simulink model "BikeRLAgent"  (R2023b)
settings: Solver=VariableStepAuto  StartTime=0.0  StopTime=inf  RelTol=1e-3
values from neighbouring files (symbols this model uses):
  angleFF = (lambda)    [config.m]
  angleRF = angleRF * (180/pi)    [config.m]
  b_contact_RW = 2e3    (= 2000)    [config.m]
  C_F_alpha = 1e3    (= 1000)    [config.m]
  C_F_kappa = 1e3    (= 1000)    [config.m]
  CM_phi = 0.3    [config.m]
  Dtheta0 = v0 / radiusRW    (= 0)    [config.m]
  Dtheta0_FW = v0 / radiusFW    (= 0)    [config.m]
  epsilon = 1e-2    (= 0.01)    [config.m]
  g = 9.81    [config.m]
  isoCameraAimX = (1/2)*w + 0.75    (= 1.267)    [config.m]
  isoCameraX = -2    [config.m]
  isoCameraY = -1.0    (= -1)    [config.m]
  isoCameraZ = -2*w    (= -2.068)    [config.m]
  k_contact_FW = 1e5    (= 100000)    [config.m]
  k_contact_RW = 1e5    (= 100000)    [config.m]
  lengthFF = frontHinge / (sind(lambda))    [config.m]
  lengthRF = sqrt((w-frontHinge)^2 + adj^2)    [config.m]
  lengthRW = 0.03    [config.m]
  massRW = 2    [config.m]
  max_cte = 7    [config.m]
  max_lean = 60    [config.m]
  max_positive_vel_error = 3    [config.m]
  max_rw_t = 20.0    (= 20)    [config.m]
  max_steer_t = 2.0    (= 2)    [config.m]
  max_steering = 70    [config.m]
  mB = 15    [config.m]
  mH = 5    [config.m]
  radiusFW = 0.325    [config.m]
  radiusRW = 0.32    [config.m]
  ref_v = ref_v_lims(1) + (ref_v_lims(2) - ref_v_lims(1))*rand(1,1)    [ResetFcn.m]
  sigma = 0.12    [config.m]
  topViewX = -4.5*w    (= -4.653)    [config.m]
  topViewY = 0*w    (= 0)    [config.m]
  topViewZ = 1*w    (= 1.034)    [config.m]
  xPla = 3e3    (= 3000)    [config.m]
  yPla = 3e3    (= 3000)    [config.m]
  zPla = 0.01    [config.m]
undefined symbols (not defined in the file or in its folder): Cylinder, Parts_Lib, ref_theta, ref_x, ref_y, X, Y, Z
libraries: sm_lib x78, nesl_utility x32, vrlib x14, simulink x6, rllib x1
(part 1 of 4)
Description:
  | Bicycle Simator was developed as a requirement for my Thesis, supervised by Alen Turnwald (MSc) at the Institute of Control Systems, TU Kaiserslautern.
  | 
  | More details on the theory can be found for the tire models at:
  | 
  | [1] De Vries , E J H. ; Den Brok , J F A.: Assessing slip of a rolling disc and the implementation of a tyre model in the benchmark bicycle. (2010), S. 20–22
  | 
  | [2] denBrok , J.F.A: A SimMechnaics Motorcycle Tyre Model for Real Time Purposes , TU Delft, Diplomarbeit
  | 
  | [3] Pacejka , H.B.: Tyre and Vehicle Dynamics.
  | 
  | [4] Maurice , J.P ; Pacejka , H.B: Relaxation length behavior of tyres. In: Vehicle System Dynamics Supplement S1 (1997), Nr. 27, S. 339–342. http://dx.doi.org/10.1080/00423119708969668. – DOI10.1080/00423119708969668
  | 
  | The bicycle modes are simulated according to:
  | 
  | [1] Meijaard , J.P. ; Papadopoulos , Jim M. ; Ruina , Andy ; Schwab , A.L.: Linearized dynamics equations for the balance and steer of a bicycle: a benchmark and review. In:
  | Proceedings of the Royal Society A: Mathematical, Physical and Engineering Sciences (2007). http://dx.doi.org/10.1098/rspa.2007.1857 . – DOI
  | 10.1098/rspa.2007.1857. – ISBN 1364–5021
  | 
  | For any suggestions or questions on the simulator, please contact me at : rzwn.hmd@gmail.com
  | 
  | For more info on the project at TU Kaiserslautern, please contact Alen through the website https://www.eit.uni-kl.de/liu/
settings Model: Creator=Rizwan Ahmed  LastModifiedBy=Asus
settings SolverCC: AlgebraicLoopSolver=TrustRegion
settings DebuggingCC: UnconnectedInputMsg=warning  UnconnectedOutputMsg=warning  UnconnectedLineMsg=warning  ArithmeticOperatorsInVariantConditions=warning
settings ModelReferenceCC: EnableRefExpFcnMdlSchedulingChecks=on
settings SFSimCC: SimUseLocalCustomCode=off  CustomCodeUndefinedFunction=UseInterfaceOnly
settings RTWCC: RTWUseLocalCustomCode=off
settings SimscapeCC: SimscapeLogType=all
settings ExplorerConfigSet: SimMechanicsOpenEditorOnUpdate=off  InternalSimMechanicsExplorerSettings="<ExplorerConfiguration><canonicalview>default</canonicalview><AnimationSetting><BasePlaybackSpeed>1.0</BasePlaybackSpeed><PlaybackSpeedFactor>1.0</PlaybackSpeedFactor></AnimationSetting><TilePanel><TileInfo><Tiles Columns=\"2\" Count=\"2\" Rows=\"1\"><Column Weight=\"0.492\"/><Column Weight=\"0.508\"/><Row Weight=\"1\"/><Tile Height=\"1\" Width=\"1\" X=\"0\" Y=\"0\"/><Tile Height=\"1\" Width=\"1\" X=\"1\" Y=\"0\"/></Tiles></TileInfo><SceneInfo><SceneViewer><BGColor><R>0.60000002384185791</R><G>0.60000002384185791</G><B>0.60000002384185791</B></BGColor><Camera><DoPerspective>on</DoPerspective><Position><X>40.0793484798167796</X><Y>-430.838153346124784</Y><Z>1.66080398163320275</Z></Position><Center><X>36.3390777502768501</X><Y>-431.839381200916819</Y><Z>0.597722304368772495</Z></Center><Up><X>0</X><Y>0</Y><Z>1</Z></Up><ViewLimDist>1</ViewLimDist><YLim>0.466307658154998583</YLim><XLim>0.306480927864584751</XLim></Camera></SceneViewer><SceneViewer><BGColor><R>0.60000002384185791</R><G>0.60000002384185791</G><B>0.60000002384185791</B></BGColor><Camera><DoPerspective>on</DoPerspective><Position><X>37.7119066108340064</X><Y>-431.61831898274437</Y><Z>5.04420073289151016</Z></Position><Center><X>36.3390777502768501</X><Y>-431.839381200916819</Y><Z>0.597722304368772495</Z></Center><Up><X>0</X><Y>0</Y><Z>1</Z></Up><ViewLimDist>1</ViewLimDist><YLim>0.466307658154998583</YLim><XLim>0.316140785189829521</XLim></Camera></SceneViewer></SceneInfo></TilePanel><MechEditorPanel><Cameras><Camera><Id>Camera1</Id><Value><Name>FollowerCAM</Name><NativeCamera><PositionTrackingFeature>env.Blue_Bike.Rear_Frame.Camera.Isometric_Camera.F</PositionTrackingFeature><CenterTrackingFeature>env.Blue_Bike.Rear_Frame.Camera.Isometric_Camera_Aim.F</CenterTrackingFeature><UpVectorTrackingFeature>env.World_Frame.W</UpVectorTrackingFeature><CenterTrackingOrigin>on</CenterTrackingOrigin><UpVectorTrackingDirection>+Z</UpVectorTrackingDirection></NativeCamera></Value></Camera><Camera><Id>Camera2</Id><Value><Name>TopViewCAM</Name><NativeCamera><PositionTrackingFeature>env.Blue_Bike.Rear_Frame.Camera.Top_View_Camera.F</PositionTrackingFeature><CenterTrackingFeature>env.Blue_Bike.Rear_Frame.Camera.Isometric_Camera_Aim.F</CenterTrackingFeature><UpVectorTrackingFeature>env.World_Frame.W</UpVectorTrackingFeature><CenterTrackingOrigin>on</CenterTrackingOrigin><UpVectorTrackingDirection>+Z</UpVectorTrackingDirection></NativeCamera></Value></Camera><Camera><Id>Camera3</Id><Value><Name>SteadyTopView</Name><NativeCamera><PositionKeyframeSet><Keyframe><Time>2.5891308412809746</Time><Value><X>-1500.2422405351419</X><Y>-1.2415472177685842</Y><Z>48.238337271221212</Z></Value></Keyframe></PositionKeyframeSet><CenterKeyframeSet><Keyframe><Time>2.5891308412809746</Time><Value><X>-1470.3262819498591</X><Y>0.22735758327736777</Y><Z>0.0049745875138000883</Z></Value></Keyframe></CenterKeyframeSet><UpVectorKeyframeSet><Keyframe><Time>2.5891308412809746</Time><Value><X>0.84986878874947092</X><Y>-0.027340292059941096</Y><Z>0.526284666639248</Z></Value></Keyframe></UpVectorKeyframeSet></NativeCamera></Value></Camera></Cameras><GfxPanelCameraMap><MapElement CameraMLId=\"Camera1\" GfxPanelIndex=\"0\"/><MapElement CameraMLId=\"Camera2\" GfxPanelIndex=\"1\"/></GfxPanelCameraMap><VideoCreator><PlaybackSpeedRatio>1.0</PlaybackSpeedRatio><FrameRate>30</FrameRate><VideoFormat>Motion JPEG AVI</VideoFormat><FrameSize>auto</FrameSize></VideoCreator></MechEditorPanel></ExplorerConfiguration>"

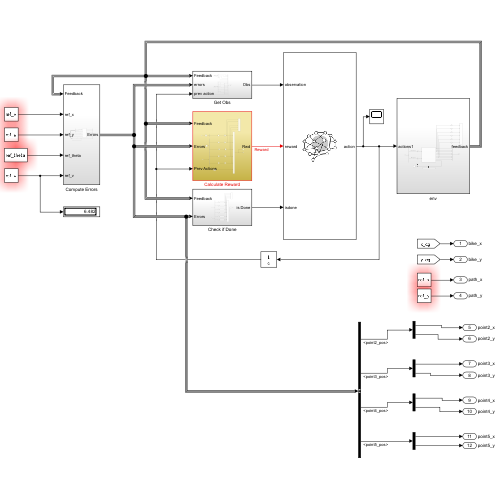
[thumbnail: Simulink's stored preview of the top-level diagram]
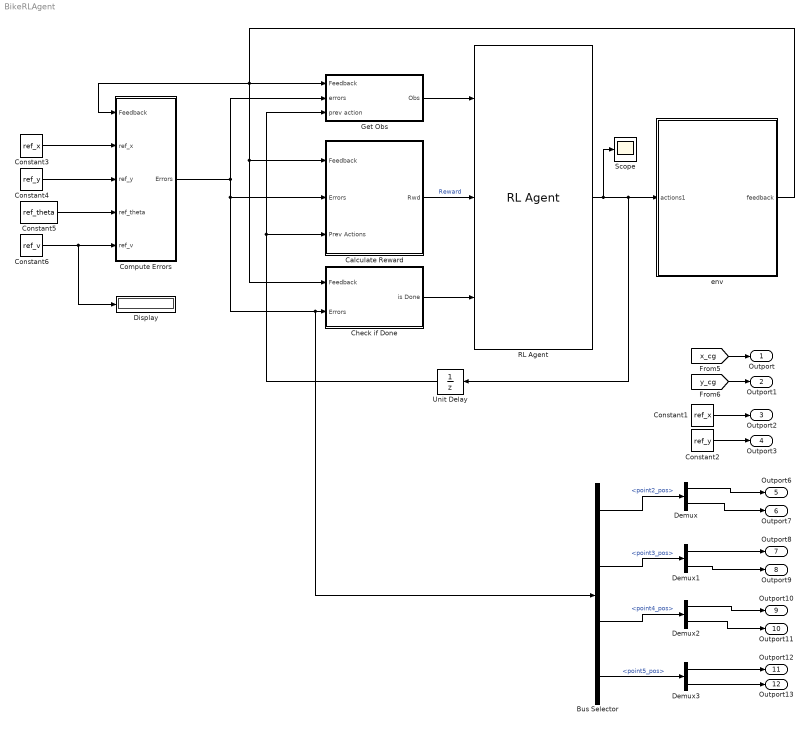
== system BikeRLAgent ==
  Bus Selector : BusSelector  OutputSignals=point2_pos,point3_pos,point4_pos,point5_pos
  Calculate Reward : Subsystem
  Check if Done : Subsystem
  Compute Errors : Subsystem
  Constant1 : Constant  Value=ref_x
  Constant2 : Constant  Value=ref_y
  Constant3 : Constant  Value=ref_x
  Constant4 : Constant  Value=ref_y
  Constant5 : Constant  Value=ref_theta
  Constant6 : Constant  Value=ref_v
  Demux{,1..3} (4 alike) : Demux  Outputs=2
  Display : Display
  Get Obs : Subsystem
  RL Agent : rllib/RL Agent  Agent=agent  ExternalActionAsInput=off  ProvideLastAction=off  ProvideCumRwd=off  TreatAsDirectFeedthrough=on  UseStrictObservationDataTypes=off
  Scope : Scope
  Unit Delay : UnitDelay  SampleTime=-1  HasFrameUpgradeWarning=on
  env : Subsystem
  Outport : Outport  SignalName=bike_x
  Outport1 : Outport  Port=2  SignalName=bike_y
  Outport2 : Outport  Port=3  SignalName=path_x
  Outport3 : Outport  Port=4  SignalName=path_y
  Outport6 : Outport  Port=5  SignalName=point2_x
  Outport7 : Outport  Port=6  SignalName=point2_y
  Outport8 : Outport  Port=7  SignalName=point3_x
  Outport9 : Outport  Port=8  SignalName=point3_y
  Outport10 : Outport  Port=9  SignalName=point4_x
  Outport11 : Outport  Port=10  SignalName=point4_y
  Outport12 : Outport  Port=11  SignalName=point5_x
  Outport13 : Outport  Port=12  SignalName=point5_y
  wires:
  [x_cg] -> Outport/1
  [y_cg] -> Outport1/1
  env/1(feedback) -> Compute Errors/1(Feedback), Get Obs/1(Feedback), Check if Done/1(Feedback), Calculate Reward/1(Feedback)
  Unit Delay/1 -> Get Obs/3(prev action), Calculate Reward/3(Prev Actions)
  Compute Errors/1(Errors) -> Calculate Reward/2(Errors), Bus Selector/1, Check if Done/2(Errors), Get Obs/2(errors)
  RL Agent/1 -> Scope/1, Unit Delay/1, env/1(actions1)
  Get Obs/1(Obs) -> RL Agent/1
  Check if Done/1(is Done) -> RL Agent/3
  Calculate Reward/1(Rwd) -> RL Agent/2  "Reward"
  Constant1/1 -> Outport2/1
  Constant2/1 -> Outport3/1
  Constant5/1 -> Compute Errors/4(ref_theta)
  Constant4/1 -> Compute Errors/3(ref_y)
  Constant3/1 -> Compute Errors/2(ref_x)
  Constant6/1 -> Display/1, Compute Errors/5(ref_v)
  Demux/2 -> Outport7/1
  Demux/1 -> Outport6/1
  Bus Selector/1 -> Demux/1  "<point2_pos>"
  Demux1/1 -> Outport8/1
  Demux1/2 -> Outport9/1
  Bus Selector/2 -> Demux1/1  "<point3_pos>"
  Bus Selector/3 -> Demux2/1  "<point4_pos>"
  Demux2/1 -> Outport10/1
  Demux2/2 -> Outport11/1
  Bus Selector/4 -> Demux3/1  "<point5_pos>"
  Demux3/1 -> Outport12/1
  Demux3/2 -> Outport13/1

== system BikeRLAgent/Calculate Reward ==
  Feedback : Inport
  Errors : Inport  Port=2
  Prev Actions : Inport  Port=3
  Abs : Abs  SaturateOnIntegerOverflow=off
  Bus Selector : BusSelector  OutputSignals=cte,velError
  Bus Selector1 : BusSelector  OutputSignals=Lean
  Demux : Demux  Outputs=2
  Duration Reward : Constant  Value=50
  Gain1 : Gain  Gain=0.5
  Gain2 : Gain  Gain=5
  Gain3 : Gain  Gain=7
  Gain4 : Gain  Gain=7
  Gain8 : Gain  Gain=5
  Rate Transition : RateTransition  OutPortSampleTime=Ts
  Rate Transition1 : RateTransition  OutPortSampleTime=Ts
  Scope : Scope  NumInputPorts=6
  Scope1 : Scope
  Square{1..3,5} (4 alike) : Math  Operator=square
  Sum : Sum  Inputs=-----+
  Rwd : Outport
  wires:
  Square1/1 -> Gain3/1
  Gain3/1 -> Scope/1, Sum/1  "Lean Reward"
  Gain2/1 -> Scope/2, Sum/2  "CTE Reward"
  Bus Selector/1 -> Abs/1  "<cte>"
  Bus Selector1/1 -> Square1/1  "<Lean>"
  Sum/1 -> Scope1/1, Rwd/1
  Square5/1 -> Gain8/1
  Demux/1 -> Square5/1  "RWTorque"
  Gain8/1 -> Scope/5, Sum/4  "RW Torque Reward"
  Rate Transition/1 -> Bus Selector1/1
  Feedback/1 -> Rate Transition/1
  Rate Transition1/1 -> Bus Selector/1
  Errors/1 -> Rate Transition1/1
  Duration Reward/1 -> Sum/6  "Duration Reward"
  Square2/1 -> Gain1/1
  Bus Selector/2 -> Square2/1  "<velError>"
  Gain1/1 -> Scope/4, Sum/3  "Velocity Reward"
  Square3/1 -> Gain4/1
  Gain4/1 -> Scope/6, Sum/5  "Steering Torque Reward"
  Demux/2 -> Square3/1  "SteeringTorque"
  Prev Actions/1 -> Demux/1
  Abs/1 -> Gain2/1

== system BikeRLAgent/Check if Done ==
  Feedback : Inport
  Errors : Inport  Port=2
  Abs{,1..3,5} (5 alike) : Abs  ZeroCross=off  SaturateOnIntegerOverflow=off
  Bus Selector : BusSelector  OutputSignals=cte,velError
  Bus Selector1 : BusSelector  OutputSignals=Position.X Coordinate,Position.Y Coordinate,Lean,Steering Angle
  Compare To Constant : simulink/Logic and Bit Operations/Compare To Constant  relop=>=  const=xPla  OutDataTypeStr=boolean
  Compare To Constant1 : simulink/Logic and Bit Operations/Compare To Constant  relop=>=  const=yPla  OutDataTypeStr=boolean  ZeroCross=off
  Compare To Constant2 : simulink/Logic and Bit Operations/Compare To Constant  relop=>=  const=max_lean * (pi/180)  OutDataTypeStr=boolean  ZeroCross=off
  Compare To Constant3 : simulink/Logic and Bit Operations/Compare To Constant  relop=>=  const=max_steering * (pi/180)  OutDataTypeStr=boolean  ZeroCross=off
  Compare To Constant4 : simulink/Logic and Bit Operations/Compare To Constant  relop=>=  const=max_cte  OutDataTypeStr=boolean  ZeroCross=off
  Compare To Constant5 : simulink/Logic and Bit Operations/Compare To Constant  relop=>=  const=max_positive_vel_error  OutDataTypeStr=boolean  ZeroCross=off
  Gain : Gain  Gain=-1
  OR : Logic  Operator=OR  Inputs=6  AllPortsSameDT=off  OutDataTypeStr=boolean
  Rate Transition : RateTransition  OutPortSampleTime=Ts
  Scope1 : Scope  NumInputPorts=6
  is Done : Outport
  wires:
  Bus Selector1/2 -> Abs1/1  "<Y Coordinate>"
  Abs1/1 -> Compare To Constant1/1
  Bus Selector1/1 -> Abs/1  "<X Coordinate>"
  Abs/1 -> Compare To Constant/1
  Feedback/1 -> Bus Selector1/1
  Compare To Constant1/1 -> Scope1/2, OR/2  "Y Coordinate Done"
  Compare To Constant/1 -> OR/1, Scope1/1  "X Coordinate Done"
  Abs2/1 -> Compare To Constant2/1
  Bus Selector1/3 -> Abs2/1  "<Lean>"
  Compare To Constant2/1 -> Scope1/3, OR/3  "Lean Done"
  Abs5/1 -> Compare To Constant3/1
  Bus Selector1/4 -> Abs5/1  "<Steering Angle>"
  Compare To Constant3/1 -> Scope1/4, OR/4  "Steering Angle Done"
  Rate Transition/1 -> is Done/1
  OR/1 -> Rate Transition/1
  Errors/1 -> Bus Selector/1
  Compare To Constant4/1 -> Scope1/5, OR/5  "CTE Done"
  Abs3/1 -> Compare To Constant4/1
  Bus Selector/1 -> Abs3/1  "<cte>"
  Compare To Constant5/1 -> Scope1/6, OR/6  "Vel Error Done"
  Bus Selector/2 -> Gain/1  "<velError>"
  Gain/1 -> Compare To Constant5/1

== system BikeRLAgent/Compute Errors ==
  Feedback : Inport
  ref_x : Inport  Port=2
  ref_y : Inport  Port=3
  ref_theta : Inport  Port=4
  ref_v : Inport  Port=5
  Bus Creator : BusCreator  Inputs=7
  Bus Selector1 : BusSelector  OutputSignals=RW Angular Velocity
  Bus Selector2 : BusSelector  OutputSignals=Position.X Coordinate,Position.Y Coordinate,Yaw
  Gain7 : Gain  Gain=radiusRW
  MATLAB Function : MATLAB Function  TreatAsAtomicUnit=on
  Matrix Concatenate : Concatenate  Mode=Multidimensional array  ConcatenateDimension=2
  Mux1 : Mux  Inputs=2
  Sum1 : Sum  Inputs=|-+
  Errors : Outport
  wires:
  MATLAB Function/1(cte) -> Bus Creator/1
  Mux1/1 -> MATLAB Function/1(bike_pos)
  Bus Selector2/2 -> Mux1/2  "<Y Coordinate>"
  MATLAB Function/2(yawError) -> Bus Creator/2
  Bus Selector2/3 -> MATLAB Function/2(bike_yaw)  "<Yaw>"
  Bus Creator/1 -> Errors/1
  Bus Selector2/1 -> Mux1/1  "<X Coordinate>"
  Matrix Concatenate/1 -> MATLAB Function/3(ref_path)
  MATLAB Function/3(point2_pos) -> Bus Creator/3
  MATLAB Function/4(point3_pos) -> Bus Creator/4
  MATLAB Function/5(point4_pos) -> Bus Creator/5
  MATLAB Function/6(point5_pos) -> Bus Creator/6
  ref_x/1 -> Matrix Concatenate/1
  ref_y/1 -> Matrix Concatenate/2
  ref_theta/1 -> MATLAB Function/4(ref_yaw)
  Feedback/1 -> Bus Selector2/1, Bus Selector1/1
  Gain7/1 -> Sum1/1  "Rear Wheel Velocity [m/s]"
  Sum1/1 -> Bus Creator/7  "velError"
  ref_v/1 -> Sum1/2
  Bus Selector1/1 -> Gain7/1  "<RW Angular Velocity>"

== system BikeRLAgent/Get Obs ==
  Feedback : Inport
  errors : Inport  Port=2
  prev action : Inport  Port=3
  Bus Selector : BusSelector  OutputSignals=Lean Rate,Lean,Steering Angle,Steering Rate
  Bus Selector1 : BusSelector  OutputSignals=cte,velError,point2_pos,point3_pos,point4_pos,point5_pos
  Demux{,1..3} (4 alike) : Demux  Outputs=2
  Mux1 : Mux  Inputs=15
  Rate Transition : RateTransition
  Rate Transition1 : RateTransition  OutPortSampleTime=Ts
  Rate Transition2 : RateTransition  OutPortSampleTime=Ts
  Obs : Outport
  wires:
  Mux1/1 -> Rate Transition/1
  Demux/1 -> Mux1/11
  Bus Selector/1 -> Mux1/1  "<Lean Rate>"
  Bus Selector/2 -> Mux1/2  "<Lean>"
  Bus Selector/3 -> Mux1/3  "<Steering Angle>"
  Bus Selector/4 -> Mux1/4  "<Steering Rate>"
  Bus Selector1/1 -> Mux1/5  "<cte>"
  Demux/2 -> Mux1/12
  Demux1/1 -> Mux1/13
  Demux1/2 -> Mux1/14
  prev action/1 -> Mux1/15
  Rate Transition/1 -> Obs/1
  Rate Transition1/1 -> Bus Selector/1
  Feedback/1 -> Rate Transition1/1
  Rate Transition2/1 -> Bus Selector1/1
  errors/1 -> Rate Transition2/1
  Demux2/1 -> Mux1/9
  Demux2/2 -> Mux1/10
  Demux3/2 -> Mux1/8
  Demux3/1 -> Mux1/7
  Bus Selector1/3 -> Demux3/1  "<point2_pos>"
  Bus Selector1/4 -> Demux2/1  "<point3_pos>"
  Bus Selector1/5 -> Demux/1  "<point4_pos>"
  Bus Selector1/6 -> Demux1/1  "<point5_pos>"
  Bus Selector1/2 -> Mux1/6  "<velError>"

== system BikeRLAgent/env ==
  note: Rear wheel torque
  note: Steering Torque
  actions1 : Inport
  Blue Bike : Subsystem
      mask Display: image('BlueBike.PNG');
  Bus Creator : BusCreator  Inputs=8
  Config : Subsystem
  Demux : Demux  Outputs=2
  Gain{,4,8..9} (4 alike) : Gain  Gain=180/pi
  Gain1 : Gain  Gain=(180/pi)
  Gain2 : Gain  Gain=radiusRW
  Plane : Subsystem  mask(Plane for SimMechanics){Parameter4=None, xPla=xPla, yPla=yPla, zPla=zPla, plane_Color=Default, grid_color=Default}
      mask prompts: xPla "Plane Length along X [m]"; yPla "Plane Length along Y [m]"; zPla "Plane depth along Z [m]"; plane_Color "Plane"; grid_color "Grids"
      mask help:
      | _______________________________________________________________________________________
      | Enter the values for the plane dimensions along {X,Y,Z} in the inertial frame.
      |
      | !! When using grids along the plane, make sure that X and Y make a square dimension.!!
      mask init:
      | curblk = gcb;
      | if strcmp(get_param(curblk,'plane_Color'),'Default')
      |     set_param([curblk '/plane'],'GraphicDiffuseColor','[0.5 0.5 0.5]');
      | elseif strcmp(get_param(gcb,'plane_Color'),'Black')
      |     set_param([curblk '/plane'],'GraphicDiffuseColor','[0.0 0.0 0.0]');
      | elseif strcmp(get_param(gcb,'plane_Color'),'White')
      |     set_param([curblk '/plane'],'GraphicDiffuseColor','[1.0 1.0 1.0]');
      | end
      | 
      | if strcmp(get_param(curblk,'grid_color'),'Default')
      |     set_param([curblk '/Grid/Grid_XLines'],'GraphicDiffuseColor','[1.0 1.0 1.0]');
      |     set_param([curblk '/Grid/Grid_YLines'],'GraphicDiffuseColor','[1.0 1.0 1.0]');
      | elseif strcmp(get_param(curblk,'grid_color'),'Black')
      |     set_param([curblk '/Grid/Grid_XLines'],'GraphicDiffuseColor','[0.0 0.0 0.0]');
      |     set_param([curblk '/Grid/Grid_YLines'],'GraphicDiffuseColor','[0.0 0.0 0.0]');
      | elseif strcmp(get_param(curblk,'grid_color'),'Grey')
      |     set_param([curblk '/Grid/Grid_XLines'],'GraphicDiffuseColor','[0.5 0.5 0.5]');
      |     set_param([curblk '/Grid/Grid_YLines'],'GraphicDiffuseColor','[0.5 0.5 0.5]');
      | end
      | clear curblk
      mask TypeOptions Parameter4: None | Grids
      mask TypeOptions plane_Color: Default | Black | White
      mask TypeOptions grid_color: Default | Black | Grey
      mask DialogControl Container3 Prompt: Color
      mask Display: image('the_road.jpg');
  Scope : Scope  NumInputPorts=6
  World Frame : sm_lib/Frames and Transforms/World Frame
  max rear wheel torque : Gain  Gain=max_rw_t
  max steering torque1 : Gain  Gain=max_steer_t
  feedback : Outport
  wires:
  Blue Bike/7(Steering Rate) -> Gain8/1, Bus Creator/7  "Steering Rate"
  Blue Bike/2(Lean) -> Gain/1, Bus Creator/2  "Lean"
  Blue Bike/1(Lean Rate) -> Bus Creator/1, Gain9/1  "Lean Rate"
  Blue Bike/5(Position) -> Bus Creator/5  "Position"
  Blue Bike/8(FW Angular Velocity) -> Bus Creator/8  "FW Angular Velociy"
  Blue Bike/6(Steering) -> Gain4/1, Bus Creator/6  "Steering Angle"
  Blue Bike/3(RW Angular Velocity) -> Bus Creator/3, Gain2/1  "RW Angular Velocity"
  Bus Creator/1 -> feedback/1
  Gain2/1 -> Scope/1  "Rear Wheel Velocity [m/s]"
  Gain4/1 -> Scope/6  "Steering Angle [deg]"
  Blue Bike/4(Yaw) -> Gain1/1, Bus Creator/4  "Yaw"
  Gain/1 -> Scope/3  "Lean  [deg]"
  Gain8/1 -> Scope/5  "Steering Rate [deg/s]"
  Gain9/1 -> Scope/2  "Lean Rate [deg/s]"
  Gain1/1 -> Scope/4  "Orientation [deg]"
  Demux/2 -> max steering torque1/1
  max rear wheel torque/1 -> Blue Bike/1(Cycling Toque)
  actions1/1 -> Demux/1
  max steering torque1/1 -> Blue Bike/2(Steering Torque)
  Demux/1 -> max rear wheel torque/1
  connections:
  Config/RConn1 -- Blue Bike/RConn1 -- Plane/LConn1 -- World Frame/RConn1

== system BikeRLAgent/env/Blue Bike ==
  Cycling Toque : Inport
  Steering Torque : Inport  Port=2
  Front Axle : sm_lib/Joints/Revolute Joint  JointMode=Normal  SenseConstraintForce=off  SenseConstraintForceX=off  SenseConstraintForceY=off  SenseConstraintForceZ=off  SenseConstraintTorque=off  SenseConstraintTorqueX=off  SenseConstraintTorqueY=off  SenseConstraintTorqueZ=off  SenseTotalForce=off  SenseTotalForceX=off  SenseTotalForceY=off  SenseTotalForceZ=off  SenseTotalTorque=off  SenseTotalTorqueX=off  SenseTotalTorqueY=off  SenseTotalTorqueZ=off  CompositeWrenchDir=FollowerOnBase  CompositeWrenchFrame=BaseFrame  EquilibriumPosition=0  EquilibriumPositionUnits=deg  SpringStiffness=0  SpringStiffnessUnits=N*m/deg  DampingCoefficient=0  DampingCoefficientUnits=N*m/(deg/s)  TorqueActuationMode=NoTorque  MotionActuationMode=ComputedMotion  SensePosition=off  SenseVelocity=off  SenseAcceleration=off  SenseTorqueForce=off  SenseLowerLimitTorqueForce=off  SenseUpperLimitTorqueForce=off  LowerLimitSpecify=off  LowerLimitBound=-90  LowerLimitBoundUnits=deg  LowerLimitStiffness=1e4  LowerLimitStiffnessUnits=N*m/deg  LowerLimitDamping=10  LowerLimitDampingUnits=N*m/(deg/s)  LowerLimitTransitionRegionWidth=0.1  LowerLimitTransitionRegionWidthUnits=deg  UpperLimitSpecify=off  UpperLimitBound=90  UpperLimitBoundUnits=deg  UpperLimitStiffness=1e4  UpperLimitStiffnessUnits=N*m/deg  UpperLimitDamping=10  UpperLimitDampingUnits=N*m/(deg/s)  UpperLimitTransitionRegionWidth=0.1  UpperLimitTransitionRegionWidthUnits=deg  PositionTargetSpecify=off  PositionTargetPriority=High  PositionTargetValue=0  PositionTargetValueUnits=deg  VelocityTargetSpecify=off  VelocityTargetPriority=High  VelocityTargetValue=0  VelocityTargetValueUnits=deg/s
  Front Frame : Subsystem
      mask Display: image('BikeFrontFrame.PNG');
  Front Wheel : Subsystem  mask{radius=radiusFW, lengthFW=lengthRW, mass=massRW, k_contact=k_contact_FW, b_contact=b_contact_RW, C_F_kappa=C_F_kappa, C_F_alpha=C_F_alpha, CM_phi=CM_phi, sigma=sigma}
      mask prompts: radius "Radius [m]"; lengthFW "Thickness [m]"; mass "Mass [m]"; k_contact "Comtact Stiffness (N/m)"; b_contact "Contact Damping (N/m-s)"; C_F_kappa "Longitudinal Stiffness (N/m)"; C_F_alpha "Lateral Stiffness (N/m)"; CM_phi "Self-Aligining Stiffness (N-m/rad)"; sigma "Relaxation Length (m)"
      mask DialogControl Container4 Prompt: Geometry
      mask DialogControl Container5 Prompt: Tire parameters
      mask Display: image('BikeWheel.PNG');
  Handlebar : Subsystem
      mask Display: image('BikeSteeringHead.PNG');
  Rear Axle : sm_lib/Joints/Revolute Joint  JointMode=Normal  SenseConstraintForce=off  SenseConstraintForceX=off  SenseConstraintForceY=off  SenseConstraintForceZ=off  SenseConstraintTorque=off  SenseConstraintTorqueX=off  SenseConstraintTorqueY=off  SenseConstraintTorqueZ=off  SenseTotalForce=off  SenseTotalForceX=off  SenseTotalForceY=off  SenseTotalForceZ=off  SenseTotalTorque=off  SenseTotalTorqueX=off  SenseTotalTorqueY=off  SenseTotalTorqueZ=off  CompositeWrenchDir=FollowerOnBase  CompositeWrenchFrame=BaseFrame  EquilibriumPosition=0  EquilibriumPositionUnits=deg  SpringStiffness=0  SpringStiffnessUnits=N*m/deg  DampingCoefficient=0  DampingCoefficientUnits=N*m/(deg/s)  TorqueActuationMode=NoTorque  MotionActuationMode=ComputedMotion  SensePosition=off  SenseVelocity=off  SenseAcceleration=off  SenseTorqueForce=off  SenseLowerLimitTorqueForce=off  SenseUpperLimitTorqueForce=off  LowerLimitSpecify=off  LowerLimitBound=-90  LowerLimitBoundUnits=deg  LowerLimitStiffness=1e4  LowerLimitStiffnessUnits=N*m/deg  LowerLimitDamping=10  LowerLimitDampingUnits=N*m/(deg/s)  LowerLimitTransitionRegionWidth=0.1  LowerLimitTransitionRegionWidthUnits=deg  UpperLimitSpecify=off  UpperLimitBound=90  UpperLimitBoundUnits=deg  UpperLimitStiffness=1e4  UpperLimitStiffnessUnits=N*m/deg  UpperLimitDamping=10  UpperLimitDampingUnits=N*m/(deg/s)  UpperLimitTransitionRegionWidth=0.1  UpperLimitTransitionRegionWidthUnits=deg  PositionTargetSpecify=off  PositionTargetPriority=High  PositionTargetValue=0  PositionTargetValueUnits=deg  VelocityTargetSpecify=off  VelocityTargetPriority=High  VelocityTargetValue=0  VelocityTargetValueUnits=deg/s
  Rear Frame : Subsystem
      mask Display: image('BikeRearFrame.PNG');
  Rear Wheel : Subsystem  mask{radius=radiusRW, lengthRW=lengthRW, mass=massRW, k_contact=k_contact_RW, b_contact=b_contact_RW, C_F_kappa=C_F_kappa, C_F_alpha=C_F_alpha, CM_phi=CM_phi, sigma=sigma}
      mask prompts: radius "radius [m]"; lengthRW "thickness [m]"; mass "mass [kg]"; k_contact "Contact Stiffness (N/m)"; b_contact "Contact Damping (N/m-s)"; C_F_kappa "Longitudinal Stiffness (N/m)"; C_F_alpha "Lateral Stiffness (N/m)"; CM_phi "Self-Aligining Stiffness (N-m/rad)"; sigma "Relaxation Length (m)"
      mask DialogControl Container4 Prompt: Geomtery
      mask DialogControl Container5 Prompt: Tire parameters
      mask Display: image('BikeWheel.PNG');
  Plane : PMIOPort  Side=Right
  Lean Rate : Outport  VectorParamsAs1DForOutWhenUnconnected=off
  Lean : Outport  Port=2  VectorParamsAs1DForOutWhenUnconnected=off
  RW Angular Velocity : Outport  Port=3  VectorParamsAs1DForOutWhenUnconnected=off
  Yaw : Outport  Port=4  VectorParamsAs1DForOutWhenUnconnected=off
  Position : Outport  Port=5  VectorParamsAs1DForOutWhenUnconnected=off
  Steering : Outport  Port=6  VectorParamsAs1DForOutWhenUnconnected=off
  Steering Rate : Outport  Port=7  VectorParamsAs1DForOutWhenUnconnected=off
  FW Angular Velocity : Outport  Port=8  VectorParamsAs1DForOutWhenUnconnected=off
  wires:
  Rear Wheel/3(RW Angular Velocity) -> RW Angular Velocity/1
  Cycling Toque/1 -> Rear Wheel/1(T_phi)
  Front Wheel/1(omegaFW) -> FW Angular Velocity/1
  Rear Wheel/2(Lean) -> Lean/1
  Steering Torque/1 -> Handlebar/1(T_delta)
  Handlebar/1(delta) -> Steering/1
  Handlebar/2(Ddelta) -> Steering Rate/1
  Rear Wheel/1(Lean Rate) -> Lean Rate/1
  Rear Wheel/5(Position) -> Position/1
  Rear Wheel/4(Yaw) -> Yaw/1
  connections:
  Rear Wheel/RConn1 -- Rear Axle/RConn1
  Rear Frame/LConn1 -- Rear Axle/LConn1
  Rear Wheel/LConn1 -- Front Wheel/LConn1 -- Plane/RConn1
  Front Axle/RConn1 -- Front Wheel/RConn1
  Front Frame/LConn1 -- Front Axle/LConn1
  Rear Frame/RConn1 -- Handlebar/LConn1
  Front Frame/RConn1 -- Handlebar/RConn1

== system BikeRLAgent/env/Config ==
  Mechanism Configuration : sm_lib/Utilities/Mechanism Configuration  UniformGravity=Constant  GravityVector=[0 0 -g]  GravityVectorUnits=m/s^2  LinearizationDelta=0.001  JointModeTransitionNonlinearIterations=2
  Solver Configuration : nesl_utility/Solver Configuration  PhysicalDomain=network_engine_domain  SubClassName=solver  LeftPortType=input  RightPortType=generic  Tones=[]  Harmonics=[]  SimulateNoise=off  Profile=off  UseLocalSampling=off  EnableSwitchedLinearOptims=on  FrequencyDomain=off  UseCCode=off  RelTol=0.001  AbsTol=1e-06  MinStep=1e-09  ToWorkspace=off  RevertToSquareIcSolve=off  NumHomotopyIterations=100  PhasorMode=off  PhasorModeNumHarmonics=1  ConsistencySolver=NEWTON_FTOL  IndexReductionMethod=DerivativeReplacement  DoDC=off  ResidualTolerance=1e-09  ConsistencyTolSource=GLOBAL  ConsistencyAbsTol=0.001  ConsistencyRelTol=0.001  ConsistencyTolFactor=0.001  UseLocalSolver=off  LocalSolverChoice=NE_BACKWARD_EULER_ADVANCER  ResolveIndetEquations=on  FunctionEvalNumThread=1  LocalSolverSampleTime=0.001  DoFixedCost=off  MaxNonlinIter=3  MaxModeIter=2  ComputeImpulses=off  ImpulseIterations=2  LinearAlgebra=Sparse  LinearAlgebraNumThread=0  EquationFormulation=NE_TIME_EF  DelaysMemoryBudget=1024  AutomaticFiltering=on  FilteringTimeConstant=0.001  PartitionStorageMethod=AS_NEEDED  PartitionMemoryBudget=1024  PartitionMethod=FAST  MultibodyUseLocalSolver=off  MultibodyLocalSolverChoice=ODE1  MultibodyLocalSolverSampleTime=0.001
  C : PMIOPort  Side=Right
  connections:
  C/RConn1 -- Mechanism Configuration/RConn1 -- Solver Configuration/RConn1

== system BikeRLAgent/env/Plane ==
  note: Ground Plane
  Grid : Subsystem
  plane : sm_lib/Body Elements/Brick Solid  GraphicAmbientColor=[0.15 0.15 0.15 1.0]  BasedOnType=Density  BrickDimensions=[xPla yPla zPla]  BrickDimensionsUnits=m  CenterOfMass=[0 0 0]  CenterOfMassUnits=m  GraphicDiffuseColor=[0.5 0.5 0.5]  Density=1000  DensityUnits=kg/m^3  DoExposeReferenceFrame=on  GraphicEmissiveColor=[0.0 0.0 0.0 1.0]  ExportEntireGeometry=off  SerializedFrames=<Frames/>  MarkerShape=Sphere  MarkerSize=10  GraphicType=FromGeometry  InertiaType=CalculateFromGeometry  Mass=1  MassUnits=kg  MomentsOfInertia=[1 1 1]  MomentsOfInertiaUnits=kg*m^2  GraphicOpacity=0.5  ProductsOfInertia=[1 1 1]  ProductsOfInertiaUnits=kg*m^2  GraphicShininess=75  GraphicSpecularColor=[0.5 0.5 0.5 1.0]  GraphicVisPropType=SimpleVisualProperties
  Conn1 : PMIOPort  Side=Left
  connections:
  Grid/LConn1 -- Conn1/RConn1 -- plane/RConn1

== system BikeRLAgent/env/Blue Bike/Front Frame ==
  Align FF to Steer : sm_lib/Frames and Transforms/Rigid Transform  TranslationMethod=None  TranslationStandardOffset=0  TranslationStandardOffsetUnits=m  TranslationStandardAxis=+Z  TranslationCartesianOffset=[0 0 0]  TranslationCartesianOffsetUnits=m  TranslationROffset=0  TranslationROffsetUnits=m  TranslationZOffset=0  TranslationZOffsetUnits=m  TranslationThetaOffset=0  TranslationThetaOffsetUnits=deg  RotationMethod=StandardAxis  RotationAngleUnits=deg  RotationStandardAxis=+Y  RotationAngle=180  RotationArbitraryAxis=[0 0 1]  FollAlignAxisA=+X  BaseAlignAxisA=+Y  FollAlignAxisB=+Y  BaseAlignAxisB=+Z  RotationSequenceAxes=FollowerAxes  RotationSequence=XYX  RotationSequenceAngles=[0 0 0]  RotationSequenceAnglesUnits=deg  RotationMatrix=[1 0 0; 0 1 0; 0 0 1]  Quaternion=[1 0 0 0]
  Align to steer : sm_lib/Frames and Transforms/Rigid Transform  TranslationMethod=None  TranslationStandardOffset=0  TranslationStandardOffsetUnits=m  TranslationStandardAxis=+Z  TranslationCartesianOffset=[0 0 0]  TranslationCartesianOffsetUnits=m  TranslationROffset=0  TranslationROffsetUnits=m  TranslationZOffset=0  TranslationZOffsetUnits=m  TranslationThetaOffset=0  TranslationThetaOffsetUnits=deg  RotationMethod=StandardAxis  RotationAngleUnits=deg  RotationStandardAxis=-X  RotationAngle=90  RotationArbitraryAxis=[0 0 1]  FollAlignAxisA=+X  BaseAlignAxisA=+Y  FollAlignAxisB=+Y  BaseAlignAxisB=+Z  RotationSequenceAxes=FollowerAxes  RotationSequence=XYX  RotationSequenceAngles=[0 0 0]  RotationSequenceAnglesUnits=deg  RotationMatrix=[1 0 0; 0 1 0; 0 0 1]  Quaternion=[1 0 0 0]
  Angle FrontFrame : sm_lib/Frames and Transforms/Rigid Transform  TranslationMethod=None  TranslationStandardOffset=0  TranslationStandardOffsetUnits=m  TranslationStandardAxis=+Z  TranslationCartesianOffset=[0 0 0]  TranslationCartesianOffsetUnits=m  TranslationROffset=0  TranslationROffsetUnits=m  TranslationZOffset=0  TranslationZOffsetUnits=m  TranslationThetaOffset=0  TranslationThetaOffsetUnits=deg  RotationMethod=StandardAxis  RotationAngleUnits=deg  RotationStandardAxis=-Y  RotationAngle=angleFF  RotationArbitraryAxis=[0 0 1]  FollAlignAxisA=+X  BaseAlignAxisA=+Y  FollAlignAxisB=+Y  BaseAlignAxisB=+Z  RotationSequenceAxes=FollowerAxes  RotationSequence=XYX  RotationSequenceAngles=[0 0 0]  RotationSequenceAnglesUnits=deg  RotationMatrix=[1 0 0; 0 1 0; 0 0 1]  Quaternion=[1 0 0 0]
  Front Frame CAD : sm_lib/Body Elements/Cylindrical Solid  GraphicAmbientColor=[0.15 0.15 0.15 1.0]  BasedOnType=Density  CenterOfMass=CenterOfMassH_in_B  CenterOfMassUnits=m  GraphicDiffuseColor=[0.2 0.8 0.0]  CylinderLength=lengthFF  CylinderLengthUnits=m  CylinderRadius=cylFF  CylinderRadiusUnits=m  Density=1000  DensityUnits=kg/m^3  DoExposeReferenceFrame=on  GraphicEmissiveColor=[0.0 0.0 0.0 1.0]  ExportEntireGeometry=off  SerializedFrames=<Frames/>  MarkerShape=Sphere  MarkerSize=10  GraphicType=FromGeometry  InertiaType=Custom  Mass=mH  MassUnits=kg  MomentsOfInertia=momentInertiaH  MomentsOfInertiaUnits=kg*m^2  GraphicOpacity=0  ProductsOfInertia=ProductsofInertiaH  ProductsOfInertiaUnits=kg*m^2  GraphicShininess=75  GraphicSpecularColor=[0.5 0.5 0.5 1.0]  GraphicVisPropType=SimpleVisualProperties
  Front Frame CAD Model : Subsystem
  Len FF to Axle : sm_lib/Frames and Transforms/Rigid Transform  TranslationMethod=StandardAxis  TranslationStandardOffset=lengthFF/2  TranslationStandardOffsetUnits=m  TranslationStandardAxis=+Z  TranslationCartesianOffset=[0 0 0]  TranslationCartesianOffsetUnits=m  TranslationROffset=0  TranslationROffsetUnits=m  TranslationZOffset=0  TranslationZOffsetUnits=m  TranslationThetaOffset=0  TranslationThetaOffsetUnits=deg  RotationMethod=None  RotationAngleUnits=deg  RotationStandardAxis=+Z  RotationAngle=0.0  RotationArbitraryAxis=[0 0 1]  FollAlignAxisA=+X  BaseAlignAxisA=+Y  FollAlignAxisB=+Y  BaseAlignAxisB=+Z  RotationSequenceAxes=FollowerAxes  RotationSequence=XYX  RotationSequenceAngles=[0 0 0]  RotationSequenceAnglesUnits=deg  RotationMatrix=[1 0 0; 0 1 0; 0 0 1]  Quaternion=[1 0 0 0]
  Len FF to Steer : sm_lib/Frames and Transforms/Rigid Transform  TranslationMethod=StandardAxis  TranslationStandardOffset=lengthFF/2  TranslationStandardOffsetUnits=m  TranslationStandardAxis=+Z  TranslationCartesianOffset=[0 0 0]  TranslationCartesianOffsetUnits=m  TranslationROffset=0  TranslationROffsetUnits=m  TranslationZOffset=0  TranslationZOffsetUnits=m  TranslationThetaOffset=0  TranslationThetaOffsetUnits=deg  RotationMethod=None  RotationAngleUnits=deg  RotationStandardAxis=+Z  RotationAngle=0.0  RotationArbitraryAxis=[0 0 1]  FollAlignAxisA=+X  BaseAlignAxisA=+Y  FollAlignAxisB=+Y  BaseAlignAxisB=+Z  RotationSequenceAxes=FollowerAxes  RotationSequence=XYX  RotationSequenceAngles=[0 0 0]  RotationSequenceAnglesUnits=deg  RotationMatrix=[1 0 0; 0 1 0; 0 0 1]  Quaternion=[1 0 0 0]
  Steering : PMIOPort  Side=Right
  Axle : PMIOPort  Port=2  Side=Left
  connections:
  Len FF to Axle/LConn1 -- Angle FrontFrame/RConn1
  Steering/RConn1 -- Align FF to Steer/RConn1
  Align to steer/LConn1 -- Front Frame CAD Model/LConn1 -- Axle/RConn1
  Front Frame CAD/RConn1 -- Len FF to Axle/RConn1 -- Len FF to Steer/LConn1
  Align FF to Steer/LConn1 -- Len FF to Steer/RConn1
  Angle FrontFrame/LConn1 -- Align to steer/RConn1

== system BikeRLAgent/env/Blue Bike/Front Wheel ==
  6-DOF Joint1 : sm_lib/Joints/6-DOF Joint  JointMode=Normal  SenseConstraintForce=off  SenseConstraintForceX=off  SenseConstraintForceY=off  SenseConstraintForceZ=off  SenseConstraintTorque=off  SenseConstraintTorqueX=off  SenseConstraintTorqueY=off  SenseConstraintTorqueZ=off  SenseTotalForce=off  SenseTotalForceX=off  SenseTotalForceY=off  SenseTotalForceZ=off  SenseTotalTorque=off  SenseTotalTorqueX=off  SenseTotalTorqueY=off  SenseTotalTorqueZ=off  CompositeWrenchDir=FollowerOnBase  CompositeWrenchFrame=BaseFrame  PxEquilibriumPosition=0  PxEquilibriumPositionUnits=m  PxSpringStiffness=0  PxSpringStiffnessUnits=N/m  PxDampingCoefficient=0  PxDampingCoefficientUnits=N/(m/s)  PxTorqueActuationMode=NoTorque  PxMotionActuationMode=ComputedMotion  PxSensePosition=off  PxSenseVelocity=off  PxSenseAcceleration=off  PxSenseTorqueForce=off  PxSenseLowerLimitTorqueForce=off  PxSenseUpperLimitTorqueForce=off  PxLowerLimitSpecify=off  PxLowerLimitBound=-1  PxLowerLimitBoundUnits=m  PxLowerLimitStiffness=1e6  PxLowerLimitStiffnessUnits=N/m  PxLowerLimitDamping=1e3  PxLowerLimitDampingUnits=N/(m/s)  PxLowerLimitTransitionRegionWidth=1e-4  PxLowerLimitTransitionRegionWidthUnits=m  PxUpperLimitSpecify=off  PxUpperLimitBound=1  PxUpperLimitBoundUnits=m  PxUpperLimitStiffness=1e6  PxUpperLimitStiffnessUnits=N/m  PxUpperLimitDamping=1e3  PxUpperLimitDampingUnits=N/(m/s)  PxUpperLimitTransitionRegionWidth=1e-4  PxUpperLimitTransitionRegionWidthUnits=m  PxPositionTargetSpecify=off  PxPositionTargetPriority=High  PxPositionTargetValue=-xPla/2 + 0.1  PxPositionTargetValueUnits=m  PxVelocityTargetSpecify=on  PxVelocityTargetPriority=High  PxVelocityTargetValue=v0  PxVelocityTargetValueUnits=m/s  PyEquilibriumPosition=0  PyEquilibriumPositionUnits=m  PySpringStiffness=0  PySpringStiffnessUnits=N/m  PyDampingCoefficient=0  PyDampingCoefficientUnits=N/(m/s)  PyTorqueActuationMode=NoTorque  PyMotionActuationMode=ComputedMotion  PySensePosition=off  PySenseVelocity=off  PySenseAcceleration=off  PySenseTorqueForce=off  PySenseLowerLimitTorqueForce=off  PySenseUpperLimitTorqueForce=off  PyLowerLimitSpecify=off  PyLowerLimitBound=-1  PyLowerLimitBoundUnits=m  PyLowerLimitStiffness=1e6  PyLowerLimitStiffnessUnits=N/m  PyLowerLimitDamping=1e3  PyLowerLimitDampingUnits=N/(m/s)  PyLowerLimitTransitionRegionWidth=1e-4  PyLowerLimitTransitionRegionWidthUnits=m  PyUpperLimitSpecify=off  PyUpperLimitBound=1  PyUpperLimitBoundUnits=m  PyUpperLimitStiffness=1e6  PyUpperLimitStiffnessUnits=N/m  PyUpperLimitDamping=1e3  PyUpperLimitDampingUnits=N/(m/s)  PyUpperLimitTransitionRegionWidth=1e-4  PyUpperLimitTransitionRegionWidthUnits=m  PyPositionTargetSpecify=off  PyPositionTargetPriority=High  PyPositionTargetValue=0  PyPositionTargetValueUnits=m  PyVelocityTargetSpecify=off  PyVelocityTargetPriority=High  PyVelocityTargetValue=0  PyVelocityTargetValueUnits=m/s  PzEquilibriumPosition=0  PzEquilibriumPositionUnits=m  PzSpringStiffness=0  PzSpringStiffnessUnits=N/m  PzDampingCoefficient=0  PzDampingCoefficientUnits=N/(m/s)  PzTorqueActuationMode=NoTorque  PzMotionActuationMode=ComputedMotion  PzSensePosition=off  PzSenseVelocity=off  PzSenseAcceleration=off  PzSenseTorqueForce=off  PzSenseLowerLimitTorqueForce=off  PzSenseUpperLimitTorqueForce=off  PzLowerLimitSpecify=off  PzLowerLimitBound=-1  PzLowerLimitBoundUnits=m  PzLowerLimitStiffness=1e6  PzLowerLimitStiffnessUnits=N/m  PzLowerLimitDamping=1e3  PzLowerLimitDampingUnits=N/(m/s)  PzLowerLimitTransitionRegionWidth=1e-4  PzLowerLimitTransitionRegionWidthUnits=m  PzUpperLimitSpecify=off  PzUpperLimitBound=1  PzUpperLimitBoundUnits=m  PzUpperLimitStiffness=1e6  PzUpperLimitStiffnessUnits=N/m  PzUpperLimitDamping=1e3  PzUpperLimitDampingUnits=N/(m/s)  PzUpperLimitTransitionRegionWidth=1e-4  PzUpperLimitTransitionRegionWidthUnits=m  PzPositionTargetSpecify=on  PzPositionTargetPriority=High  PzPositionTargetValue=radiusFW  PzPositionTargetValueUnits=m  PzVelocityTargetSpecify=off  PzVelocityTargetPriority=High  PzVelocityTargetValue=0  PzVelocityTargetValueUnits=m/s  SphEqPosRotationMethod=None  SphEqPosRotationAngleUnits=deg  SphEqPosRotationStandardAxis=+Z  SphEqPosRotationAngle=0.0  SphEqPosRotationArbitraryAxis=[0 0 1]  SphEqPosFollAlignAxisA=+X  SphEqPosBaseAlignAxisA=+Y  SphEqPosFollAlignAxisB=+Y  SphEqPosBaseAlignAxisB=+Z  SphEqPosRotationSequenceAxes=FollowerAxes  SphEqPosRotationSequence=XYX  SphEqPosRotationSequenceAngles=[0 0 0]  SphEqPosRotationSequenceAnglesUnits=deg  SphEqPosRotationMatrix=[1 0 0; 0 1 0; 0 0 1]  SphEqPosQuaternion=[1 0 0 0]  SphSpringStiffness=0  SphSpringStiffnessUnits=N*m/deg  SphDampingCoefficient=damp  SphDampingCoefficientUnits=N*m/(rad/s)  SphActuateTorqueX=off  SphActuateTorqueY=off  SphActuateTorqueZ=off  SphActuateTorque=off  SphTorqueActuationMode=InputTorque  SphMotionActuationMode=ComputedMotion  SphActuationFrame=FollowerFrame  SphSensePosition=off  SphSenseVelocityX=off  SphSenseVelocityY=on  SphSenseVelocityZ=off  SphSenseVelocity=off  SphSenseAccelerationX=off  SphSenseAccelerationY=off  SphSenseAccelerationZ=off  SphSenseAcceleration=off  SphSenseTorqueX=off  SphSenseTorqueY=off  SphSenseTorqueZ=off  SphSenseTorqueForce=off  SphSenseLowerLimitTorqueMag=off  SphSenseUpperLimitTorqueMag=off  SphSensingFrame=FollowerFrame  SphLowerLimitSpecify=off  SphLowerLimitBound=15  SphLowerLimitBoundUnits=deg  SphLowerLimitStiffness=1e4  SphLowerLimitStiffnessUnits=N*m/deg  SphLowerLimitDamping=10  SphLowerLimitDampingUnits=N*m/(deg/s)  SphLowerLimitTransitionRegionWidth=0.1  SphLowerLimitTransitionRegionWidthUnits=deg  SphUpperLimitSpecify=off  SphUpperLimitBound=45  SphUpperLimitBoundUnits=deg  SphUpperLimitStiffness=1e4  SphUpperLimitStiffnessUnits=N*m/deg  SphUpperLimitDamping=10  SphUpperLimitDampingUnits=N*m/(deg/s)  SphUpperLimitTransitionRegionWidth=0.1  SphUpperLimitTransitionRegionWidthUnits=deg  SphPositionTargetRotationMethod=StandardAxis  SphPositionTargetRotationAngleUnits=deg  SphPositionTargetRotationStandardAxis=+X  SphPositionTargetRotationAngle=0  SphPositionTargetRotationArbitraryAxis=[0 0 1]  SphPositionTargetFollAlignAxisA=+X  SphPositionTargetBaseAlignAxisA=+Y  SphPositionTargetFollAlignAxisB=+Y  SphPositionTargetBaseAlignAxisB=+Z  SphPositionTargetRotationSequenceAxes=FollowerAxes  SphPositionTargetRotationSequence=XYX  SphPositionTargetRotationSequenceAngles=[0 0 0]  SphPositionTargetRotationSequenceAnglesUnits=deg  SphPositionTargetRotationMatrix=[1 0 0; 0 1 0; 0 0 1]  SphPositionTargetQuaternion=[1 0 0 0]  SphPositionTargetSpecify=on  SphPositionTargetPriority=High  SphVelocityTargetValue=[0 Dtheta0_FW 0]  SphVelocityTargetValueUnits=rad/s  SphVelocityTargetSpecify=on  SphVelocityTargetPriority=High  SphVelocityTargetInFollowerFrame=off
  Align Front Axle : sm_lib/Frames and Transforms/Rigid Transform  TranslationMethod=None  TranslationStandardOffset=0  TranslationStandardOffsetUnits=m  TranslationStandardAxis=+Z  TranslationCartesianOffset=[0 0 0]  TranslationCartesianOffsetUnits=m  TranslationROffset=0  TranslationROffsetUnits=m  TranslationZOffset=0  TranslationZOffsetUnits=m  TranslationThetaOffset=0  TranslationThetaOffsetUnits=deg  RotationMethod=StandardAxis  RotationAngleUnits=deg  RotationStandardAxis=+X  RotationAngle=90  RotationArbitraryAxis=[0 0 1]  FollAlignAxisA=+X  BaseAlignAxisA=+Y  FollAlignAxisB=+Y  BaseAlignAxisB=+Z  RotationSequenceAxes=FollowerAxes  RotationSequence=XYX  RotationSequenceAngles=[0 0 0]  RotationSequenceAnglesUnits=deg  RotationMatrix=[1 0 0; 0 1 0; 0 0 1]  Quaternion=[1 0 0 0]
  FrontTyre CAD Model : Subsystem
  PS-Simulink Converter : nesl_utility/PS-Simulink Converter  PhysicalDomain=network_engine_domain  SubClassName=ps_output  LeftPortType=input  RightPortType=output  PseudoPeriodic=off  Frequencies=[]  VectorFormat=1-D array  Unit=1  AffineConversion=off
  Tyre model FW : Subsystem
  Wheel1 : Subsystem  Tag=CustomStyle  AncestorBlock=Parts_Lib/Cylinder  mask(Solid Cylinder with Markings){cyl_radius=radiusFW, cyl_length=lengthFW, cyl_density=1000, cyl_color=red, cyl_opacity=0, cyl_color_custom=[0.7920    0.9900    0.9900], mark_radius=[0.75 0.5], mark_len_factor=1.01, mark_angle=60, mark_color=purple, mark_opacity=0}
      mask prompts: cyl_radius "Radius (m)"; cyl_length "Length (m)"; cyl_density "Density (kg/m^3)"; cyl_color "Color"; cyl_opacity "Opacity (0-1)"; cyl_color_custom "Custom Color (rgb)"; mark_radius "Outer, inner radius (% of cylinder radius)"; mark_len_factor "Length (factor of cylinder length)"; mark_angle "Sweep angle (deg)"; mark_color "Color"; mark_opacity "Opacity (0-1)"
      mask init:
      | curblk = gcb;
      | if strcmp(get_param(curblk,'cyl_color'),'red')
      |     set_param([curblk '/Cylinder'],'GraphicDiffuseColor','[0.8 0.0 0.2]');
      |     set_param(curblk,'BackGroundColor','[0.901961, 0.396078, 0.396078]');
      | elseif strcmp(get_param(gcb,'cyl_color'),'blue')
      |     set_param([curblk '/Cylinder'],'GraphicDiffuseColor','[0.0 0.5 0.7]');
      |     set_param(curblk,'BackGroundColor','[0.541176, 0.698039, 0.901961]');
      | elseif strcmp(get_param(gcb,'cyl_color'),'yellow')
      |     set_param([curblk '/Cylinder'],'GraphicDiffuseColor','[1.0 1.0 0.0]');
      |     set_param(curblk,'BackGroundColor','[0.905882, 0.890196, 0.392157]');
      | elseif strcmp(get_param(gcb,'cyl_color'),'gray')
      |     set_param([curblk '/Cylinder'],'GraphicDiffuseColor','[1.0 1.0 1.0]*0.6');
      |     set_param(curblk,'BackGroundColor','[0.6 0.6 0.6]');
      | elseif strcmp(get_param(gcb,'cyl_color'),'custom')
      |     set_param([curblk '/Cylinder'],'GraphicDiffuseColor',get_param(curblk,'cyl_color_custom'));
      |     set_param(curblk,'BackGroundColor','[1 1 1]');
      | end
      | 
      | if strcmp(get_param(curblk,'mark_color'),'purple')
      |     set_param([curblk '/Vis1'],'GraphicDiffuseColor','[0.4 0.0 0.4]');
      |     set_param([curblk '/Vis2'],'GraphicDiffuseColor','[0.4 0.0 0.4]');
      | elseif strcmp(get_param(gcb,'mark_color'),'green')
      |     set_param([curblk '/Vis1'],'GraphicDiffuseColor','[0.0 0.8 0.0]');
      |     set_param([curblk '/Vis2'],'GraphicDiffuseColor','[0.0 0.8 0.0]');
      | elseif strcmp(get_param(gcb,'mark_color'),'orange')
      |     set_param([curblk '/Vis1'],'GraphicDiffuseColor','[1.0 0.6 0.0]');
      |     set_param([curblk '/Vis2'],'GraphicDiffuseColor','[1.0 0.6 0.0]');
      | elseif strcmp(get_param(gcb,'mark_color'),'black')
      |     set_param([curblk '/Vis1'],'GraphicDiffuseColor','[0.0 0.0 0.0]');
      |     set_param([curblk '/Vis2'],'GraphicDiffuseColor','[0.0 0.0 0.0]');
      | end
      | 
      | clear curblk
      mask TypeOptions cyl_color: red | gray | yellow | blue | custom
      mask Callback cyl_color:
      | maskObj = Simulink.Mask.get(gcb);
      | clr_h = maskObj.getParameter('cyl_color_custom');
      | if strcmp(get_param(gcb,'cyl_color'),'custom')
      |     clr_h.Visible = 'on';
      | else
      |     clr_h.Visible = 'off';
      | end
      mask TypeOptions mark_color: purple | green | orange | black
      mask DialogControl Container4 Prompt: Cylinder
      mask DialogControl Container7 Prompt: Markings
  Conn4 : PMIOPort  Side=Left
  Conn5 : PMIOPort  Port=2  Side=Right
  omegaFW : Outport  VectorParamsAs1DForOutWhenUnconnected=off
  wires:
  PS-Simulink Converter/1 -> omegaFW/1
  connections:
  Align Front Axle/RConn1 -- Conn5/RConn1
  6-DOF Joint1/LConn1 -- Conn4/RConn1 -- Tyre model FW/LConn1
  6-DOF Joint1/RConn1 -- Wheel1/LConn1 -- FrontTyre CAD Model/LConn1 -- Align Front Axle/LConn1 -- Tyre model FW/RConn1
  PS-Simulink Converter/LConn1 -- 6-DOF Joint1/RConn2

== system BikeRLAgent/env/Blue Bike/Handlebar ==
  T_delta : Inport
  Gain1 : Gain  Gain=-1
  Gain2 : Gain  Gain=-1
  Handle CAD Model : Subsystem
  PS-Simulink Converter : nesl_utility/PS-Simulink Converter  PhysicalDomain=network_engine_domain  SubClassName=ps_output  LeftPortType=input  RightPortType=output  PseudoPeriodic=off  Frequencies=[]  VectorFormat=1-D array  Unit=1  AffineConversion=off
  PS-Simulink Converter1 : nesl_utility/PS-Simulink Converter  PhysicalDomain=network_engine_domain  SubClassName=ps_output  LeftPortType=input  RightPortType=output  PseudoPeriodic=off  Frequencies=[]  VectorFormat=1-D array  Unit=1  AffineConversion=off
  Simulink-PS Converter : nesl_utility/Simulink-PS Converter  PhysicalDomain=network_engine_domain  SubClassName=ps_input  LeftPortType=input  RightPortType=output  PseudoPeriodic=off  Frequencies=[]  NoiseDistribution=none  NoiseParameters=[]  Unit=1  AffineConversion=off  FilteringAndDerivatives=provide  SimscapeFilterOrder=1  InputFilterTimeConstant=0.001  UdotUserProvided=0
  Steering Joint : sm_lib/Joints/Revolute Joint  JointMode=Normal  SenseConstraintForce=off  SenseConstraintForceX=off  SenseConstraintForceY=off  SenseConstraintForceZ=off  SenseConstraintTorque=off  SenseConstraintTorqueX=off  SenseConstraintTorqueY=off  SenseConstraintTorqueZ=off  SenseTotalForce=off  SenseTotalForceX=off  SenseTotalForceY=off  SenseTotalForceZ=off  SenseTotalTorque=off  SenseTotalTorqueX=off  SenseTotalTorqueY=off  SenseTotalTorqueZ=off  CompositeWrenchDir=FollowerOnBase  CompositeWrenchFrame=BaseFrame  EquilibriumPosition=0  EquilibriumPositionUnits=deg  SpringStiffness=0  SpringStiffnessUnits=N*m/deg  DampingCoefficient=0  DampingCoefficientUnits=N*m/(deg/s)  TorqueActuationMode=InputTorque  MotionActuationMode=ComputedMotion  SensePosition=on  SenseVelocity=on  SenseAcceleration=off  SenseTorqueForce=off  SenseLowerLimitTorqueForce=off  SenseUpperLimitTorqueForce=off  LowerLimitSpecify=off  LowerLimitBound=-90  LowerLimitBoundUnits=deg  LowerLimitStiffness=1e4  LowerLimitStiffnessUnits=N*m/deg  LowerLimitDamping=10  LowerLimitDampingUnits=N*m/(deg/s)  LowerLimitTransitionRegionWidth=0.1  LowerLimitTransitionRegionWidthUnits=deg  UpperLimitSpecify=off  UpperLimitBound=90  UpperLimitBoundUnits=deg  UpperLimitStiffness=1e4  UpperLimitStiffnessUnits=N*m/deg  UpperLimitDamping=10  UpperLimitDampingUnits=N*m/(deg/s)  UpperLimitTransitionRegionWidth=0.1  UpperLimitTransitionRegionWidthUnits=deg  PositionTargetSpecify=on  PositionTargetPriority=High  PositionTargetValue=delta0  PositionTargetValueUnits=deg  VelocityTargetSpecify=off  VelocityTargetPriority=High  VelocityTargetValue=0  VelocityTargetValueUnits=deg/s
  Rear Frame : PMIOPort  Side=Left
  FrontFrame : PMIOPort  Port=2  Side=Right
  delta : Outport  VectorParamsAs1DForOutWhenUnconnected=off
  Ddelta : Outport  Port=2  VectorParamsAs1DForOutWhenUnconnected=off
  wires:
  PS-Simulink Converter/1 -> Gain1/1
  T_delta/1 -> Simulink-PS Converter/1
  Gain1/1 -> delta/1
  PS-Simulink Converter1/1 -> Gain2/1
  Gain2/1 -> Ddelta/1
  connections:
  PS-Simulink Converter1/LConn1 -- Steering Joint/RConn3
  FrontFrame/RConn1 -- Handle CAD Model/LConn1 -- Steering Joint/RConn1
  PS-Simulink Converter/LConn1 -- Steering Joint/RConn2
  Rear Frame/RConn1 -- Steering Joint/LConn1
  Steering Joint/LConn2 -- Simulink-PS Converter/RConn1
